simulink subsystem "torque_allocation"  (R2022b)
settings: Solver=VariableStepAuto  StartTime=0.0  StopTime=10.0  RelTol=1e-3
settings Model: Creator=papaveneti  LastModifiedBy=papaveneti

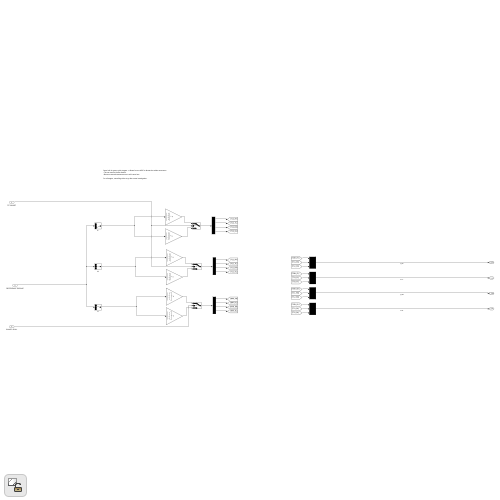
[thumbnail: Simulink's stored preview of the top-level diagram]
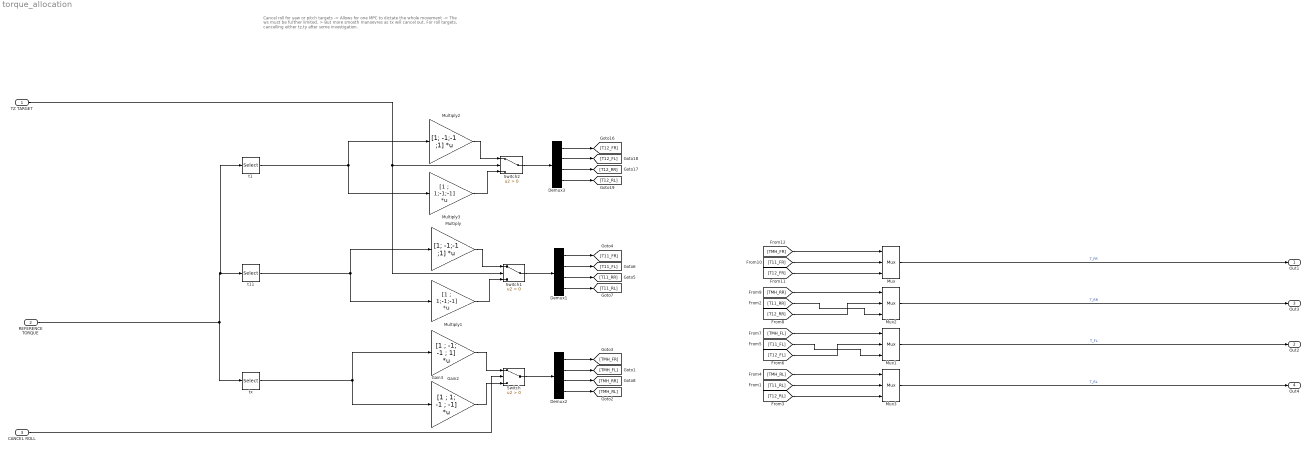
== system torque_allocation ==
  note: Cancel roll for yaw or pitch targets -> Allows for one MPC to dictate the whole movement -> The ws must be further limited.
      | > But more smooth manoevres as tx will cancel out.
      |
      | For roll targets, cancelling either tz,ty after some investigation.
  TZ TARGET : Inport
  REFERENCE TORQUE : Inport  Port=2
  CANCEL ROLL : Inport  Port=3
  Demux1 : Demux
  Demux2 : Demux
  Demux3 : Demux
  Gain2 : Gain  Gain=[1 ; -1; -1 ; 1]  Multiplication=Matrix(K*u)
  Gain3 : Gain  Gain=[1 ; 1; -1 ; -1]  Multiplication=Matrix(K*u)
  Multiply : Gain  Gain=[1; -1;-1 ;1]  Multiplication=Matrix(K*u)
  Multiply1 : Gain  Gain=[1 ; 1;-1;-1]  Multiplication=Matrix(K*u)
  Multiply2 : Gain  Gain=[1; -1;-1 ;1]  Multiplication=Matrix(K*u)
  Multiply3 : Gain  Gain=[1 ; 1;-1;-1]  Multiplication=Matrix(K*u)
  Mux{,1..3} (4 alike) : Mux  Inputs=3
  Switch : Switch  Criteria=u2 > Threshold  SaturateOnIntegerOverflow=off  InputSameDT=off
  Switch1 : Switch  Criteria=u2 > Threshold  SaturateOnIntegerOverflow=off  InputSameDT=off
  Switch2 : Switch  Criteria=u2 > Threshold  SaturateOnIntegerOverflow=off  InputSameDT=off
  t1 : Selector  InputPortWidth=3  IndexOptions=Index vector (dialog)  Indices=[3]  OutputSizes=1
  t11 : Selector  InputPortWidth=3  IndexOptions=Index vector (dialog)  Indices=[2]  OutputSizes=1
  tx : Selector  InputPortWidth=3  IndexOptions=Index vector (dialog)  Indices=1  OutputSizes=1
  Out1 : Outport
  Out2 : Outport  Port=2
  Out3 : Outport  Port=3
  Out4 : Outport  Port=4
  wires:
  CANCEL ROLL/1 -> Switch/2
  Mux2/1 -> Out3/1  "T_RR"
  Mux/1 -> Out1/1  "T_FR"
  Gain2/1 -> Switch/1
  REFERENCE TORQUE/1 -> t11/1, t1/1, tx/1
  Mux3/1 -> Out4/1  "T_RL"
  Mux1/1 -> Out2/1  "T_FL"
  tx/1 -> Gain3/1, Gain2/1
  Gain3/1 -> Switch/3
  Multiply/1 -> Switch1/1
  Switch1/1 -> Demux1/1
  Switch/1 -> Demux2/1
  Multiply1/1 -> Switch1/3
  t11/1 -> Multiply/1, Multiply1/1
  t1/1 -> Multiply3/1, Multiply2/1
  Multiply3/1 -> Switch2/3
  Switch2/1 -> Demux3/1
  Multiply2/1 -> Switch2/1
  TZ TARGET/1 -> Switch2/2, Switch1/2
  Demux1/4 -> [T11_RL]
  Demux1/2 -> [T11_FL]
  Demux1/3 -> [T11_RR]
  Demux1/1 -> [T11_FR]
  [TMH_RL] -> Mux3/1
  [TMH_FL] -> Mux1/1
  [TMH_RR] -> Mux2/1
  [T11_FR] -> Mux/2
  [T12_FR] -> Mux/3
  [TMH_FR] -> Mux/1
  Demux3/4 -> [T12_RL]
  Demux3/2 -> [T12_FL]
  Demux3/3 -> [T12_RR]
  Demux3/1 -> [T12_FR]
  Demux2/1 -> [TMH_FR]
  Demux2/2 -> [TMH_FL]
  Demux2/3 -> [TMH_RR]
  Demux2/4 -> [TMH_RL]
  [T12_RR] -> Mux2/2
  [T11_RR] -> Mux2/3
  [T12_FL] -> Mux1/2
  [T11_FL] -> Mux1/3
  [T11_RL] -> Mux3/2
  [T12_RL] -> Mux3/3
